simulink model "DUFFING"  (R2017b)
settings: Solver=VariableStepAuto  StartTime=0.0  StopTime=300.0  RelTol=1e-3
libraries: simulink x1
settings Model: Creator=DNI 53837872  LastModifiedBy=DNI 53837872
settings DataIOCC: Refine=5

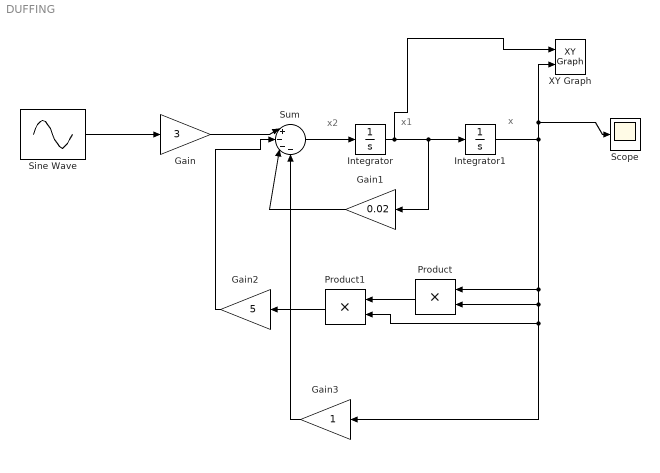
== system DUFFING ==
  note: x1
  note: x2
  note: x
  Gain : Gain  Gain=3
  Gain1 : Gain  Gain=0.02
  Gain2 : Gain  Gain=5
  Gain3 : Gain
  Integrator : Integrator
  Integrator1 : Integrator
  Product : Product
  Product1 : Product
  Scope : Scope
  Sine Wave : Sin  Frequency=0.5  SampleTime=0
  Sum : Sum  Inputs=|+---
  XY Graph : simulink/Sinks/XY Graph  xmin=-3  xmax=3  ymin=-2  ymax=2  st=-1
  wires:
  Sine Wave/1 -> Gain/1
  Gain/1 -> Sum/1
  Integrator/1 -> Integrator1/1, Gain1/1, XY Graph/1
  Integrator1/1 -> XY Graph/2, Scope/1, Product/1, Product1/2, Gain3/1, Product/2
  Gain1/1 -> Sum/3
  Product/1 -> Product1/1
  Product1/1 -> Gain2/1
  Gain2/1 -> Sum/2
  Gain3/1 -> Sum/4
  Sum/1 -> Integrator/1
